simulink model "projectCopy"  (R2018b)
settings: Solver=FixedStepAuto  StartTime=0.0  StopTime=100  FixedStep=1  RelTol=1e-3
settings Model: Creator=computer  LastModifiedBy=computer

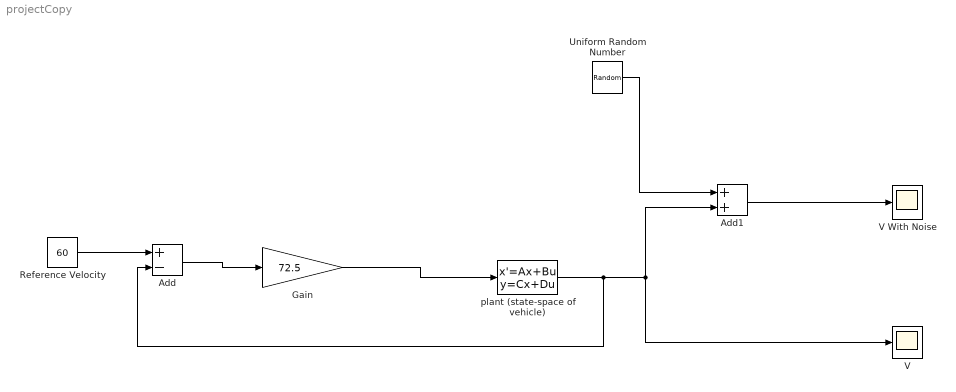
== system projectCopy ==
  Add : Sum  Inputs=+-
  Add1 : Sum
  Gain : Gain  Gain=72.5
  Reference Velocity : Constant  Value=60  SampleTime=1
  Uniform Random Number : UniformRandomNumber  Minimum=-10  Maximum=10  SampleTime=1
  V : Scope
  V With Noise : Scope
  plant (state-space of vehicle) : StateSpace  A=-50/1000  B=1/50  C=[1]  D=0  InitialCondition=0
  wires:
  Uniform Random Number/1 -> Add1/1
  Reference Velocity/1 -> Add/1
  plant (state-space of vehicle)/1 -> Add1/2, V/1, Add/2
  Add1/1 -> V With Noise/1
  Gain/1 -> plant (state-space of vehicle)/1
  Add/1 -> Gain/1
